simulink model "test_4_sim"  (R2019b)
settings: Solver=VariableStepAuto  StartTime=0.0  StopTime=15  RelTol=1e-3
values from neighbouring files (symbols this model uses):
  A = [0 1 0 0; 68747/250 0 -29463/250 0; 0 0 0 1;-19642/125 0 9821/125 0]    [test_2.m]    (also in test_3.m = [0 1 0 0; 35856471/2703500 0 -2857911/1081400 0; 0 0 0 1;-98; test_4.m = subs(jacobian(x1, x),[te,te1,a,a1,OA,AB,mB,g],x_equi); test_5.m = [0 1 0 0; 9821/750 0 -9821/2250 0; 0 0 0 1;0 0 9821/375 0]; unicycle.m = [0 1 0 0; 0 0 0 0; 0 0 0 1;0 0 5588149/150160 0])
  B = [0; -16/15; 0; 16/15]    [test_2.m]    (also in test_3.m = [0; -2250/5407; 0; 6925/5407]; test_4.m = subs(jacobian(x1, sym('M')),[te,te1,a,a1,OA,AB,mB,g],x_equi); test_5.m = [0;  -8/15; 0; 8/5]; unicycle.m = [0;  6250/17; 0; -12500/1877])
  K = place(A,B,eigs)    [test_2.m]    (also in test_3.m; test_4.m; unicycle.m = acker(A,B,eigs); unicycle_fro.m = place(A,B,eigs1))
settings Model: Creator=DooDooDude  LastModifiedBy=DooDooDude

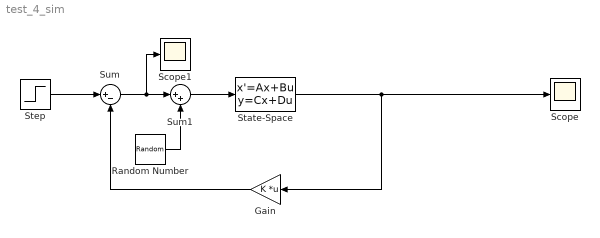
== system test_4_sim ==
  Gain : Gain  Gain=K  Multiplication=Matrix(K*u)
  Random Number : RandomNumber  Variance=0  SampleTime=0.01
  Scope : Scope
  Scope1 : Scope
  State-Space : StateSpace  A=A  B=B  C=eye(4)  D=[0; 0; 0; 0]  InitialCondition=0
  Step : Step  After=0  SampleTime=0
  Sum : Sum  Inputs=|+-
  Sum1 : Sum  Inputs=|++
  wires:
  Step/1 -> Sum/1
  Gain/1 -> Sum/2
  State-Space/1 -> Gain/1, Scope/1
  Sum/1 -> Scope1/1, Sum1/1
  Sum1/1 -> State-Space/1
  Random Number/1 -> Sum1/2
